simulink model "shemam"  (R2021a)
settings: Solver=VariableStepAuto  StartTime=0.0  StopTime=10.0  RelTol=1e-3
libraries: simulink x1
settings Model: Creator=vikau  LastModifiedBy=vikau

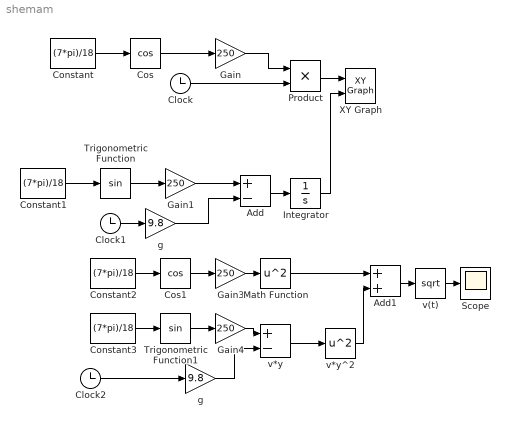
== system shemam ==
  Add : Sum  Inputs=+-
  Add1 : Sum
  Clock : Clock
  Clock1 : Clock
  Clock2 : Clock
  Constant{,1..3} (4 alike) : Constant  Value=(7*pi)/18
  Cos : Trigonometry  Operator=cos
  Cos1 : Trigonometry  Operator=cos
  Gain{,1,3..4} (4 alike) : Gain  Gain=250
  Integrator : Integrator
  Math Function : Math  Operator=square  SaturateOnIntegerOverflow=on
  Product : Product
  Scope : Scope
  Trigonometric Function : Trigonometry
  Trigonometric Function1 : Trigonometry
  XY Graph : simulink/Sinks/XY Graph  xmin=0  xmax=10000  ymin=0  ymax=3000  st=0.1
  g : Gain  Gain=9.8
  "g " : Gain  Gain=9.8
  v(t) : Sqrt  SaturateOnIntegerOverflow=on
  v*y : Sum  Inputs=+-
  v*y^2 : Math  Operator=square  SaturateOnIntegerOverflow=on
  wires:
  Constant/1 -> Cos/1
  Cos/1 -> Gain/1
  Gain/1 -> Product/1
  Clock/1 -> Product/2
  Product/1 -> XY Graph/1
  Constant1/1 -> Trigonometric Function/1
  Trigonometric Function/1 -> Gain1/1
  Gain1/1 -> Add/1
  Clock1/1 -> "g "/1
  "g "/1 -> Add/2
  Add/1 -> Integrator/1
  Integrator/1 -> XY Graph/2
  Constant2/1 -> Cos1/1
  Cos1/1 -> Gain3/1
  Gain3/1 -> Math Function/1
  Math Function/1 -> Add1/1
  Add1/1 -> v(t)/1
  v(t)/1 -> Scope/1
  Constant3/1 -> Trigonometric Function1/1
  Trigonometric Function1/1 -> Gain4/1
  Gain4/1 -> v*y/1
  v*y/1 -> v*y^2/1
  v*y^2/1 -> Add1/2
  Clock2/1 -> g/1
  g/1 -> v*y/2
